simulink model "Example4_Reading_And_Logging_Sensor_Data"  (R2016a)
settings: configuration reference "AR_Drone_ConfigSet" (kept outside this file)
libraries: AR_Drone_Sensors x2
settings Model: SimulationMode=external  Creator=sannem  LastModifiedBy=sannem
settings ConfigSetRef: SourceLocation=Base Workspace

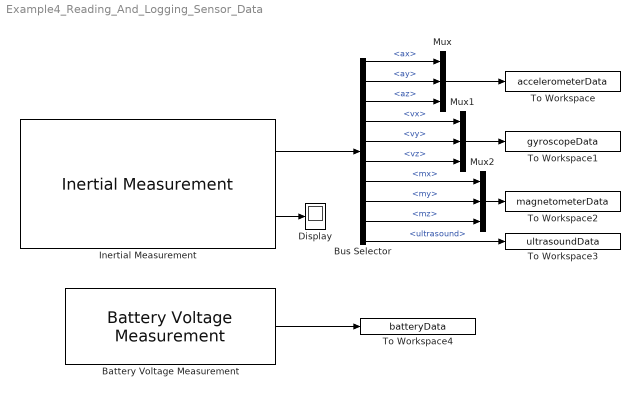
== system Example4_Reading_And_Logging_Sensor_Data ==
  Battery Voltage Measurement : AR_Drone_Sensors/Battery Voltage Measurement  SFunctionSpec=void BatteryMeasure_step(single y1[1])  SampleTime=-1
  Bus Selector : BusSelector  OutputSignals=ax,ay,az,vx,vy,vz,mx,my,mz,ultrasound
  Display : Display
  Inertial Measurement : AR_Drone_Sensors/Inertial Measurement  Ts=1/50
  Mux : Mux  Inputs=3
  Mux1 : Mux  Inputs=3
  Mux2 : Mux  Inputs=3
  To Workspace : ToWorkspace  VariableName=accelerometerData  SaveFormat=Structure With Time  SampleTime=-1
  To Workspace1 : ToWorkspace  VariableName=gyroscopeData  SaveFormat=Structure With Time  SampleTime=-1
  To Workspace2 : ToWorkspace  VariableName=magnetometerData  SaveFormat=Structure With Time  SampleTime=-1
  To Workspace3 : ToWorkspace  VariableName=ultrasoundData  SaveFormat=Structure With Time  SampleTime=-1
  To Workspace4 : ToWorkspace  VariableName=batteryData  SaveFormat=Structure With Time  SampleTime=-1
  wires:
  Mux/1 -> To Workspace/1
  Mux1/1 -> To Workspace1/1
  Mux2/1 -> To Workspace2/1
  Inertial Measurement/2 -> Display/1
  Inertial Measurement/1 -> Bus Selector/1
  Bus Selector/1 -> Mux/1  "<ax>"
  Bus Selector/2 -> Mux/2  "<ay>"
  Bus Selector/3 -> Mux/3  "<az>"
  Bus Selector/5 -> Mux1/2  "<vy>"
  Bus Selector/6 -> Mux1/3  "<vz>"
  Bus Selector/8 -> Mux2/2  "<my>"
  Bus Selector/9 -> Mux2/3  "<mz>"
  Bus Selector/7 -> Mux2/1  "<mx>"
  Bus Selector/4 -> Mux1/1  "<vx>"
  Bus Selector/10 -> To Workspace3/1  "<ultrasound>"
  Battery Voltage Measurement/1 -> To Workspace4/1
